simulink model "EFPR_HPT"  (R2024a)
settings: Solver=VariableStepAuto  StartTime=0.0  StopTime=inf  RelTol=1e-3
undefined symbols (not defined in the file): CR, LF
libraries: instrumentseriallib x2, slrealtimeseriallib x1
settings Model: Creator=enrea  LastModifiedBy=enrea

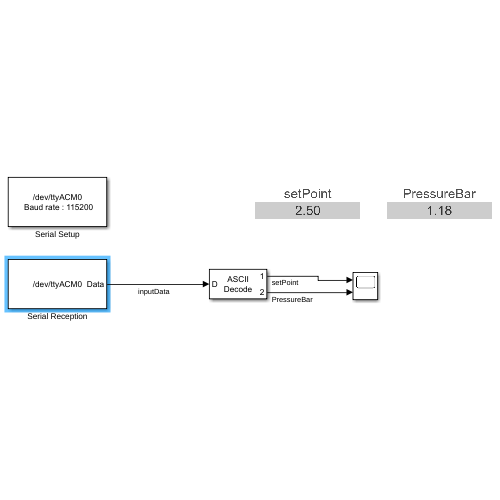
[thumbnail: Simulink's stored preview of the top-level diagram]
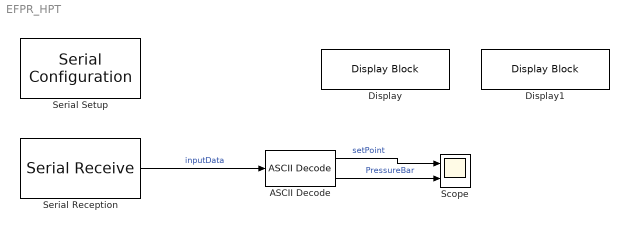
== system EFPR_HPT ==
  ASCII Decode : slrealtimeseriallib/ASCII Decode  format=%f|%f  nvars=2  vartypes={ }
  Display : DisplayBlock  Format=Custom  Transparency=1  FormatString=%.2f
  Display1 : DisplayBlock  Format=Custom  Transparency=1  FormatString=%.2f
  Scope : Scope  NumInputPorts=2
  Serial Reception : instrumentseriallib/Serial Receive  PortSel=/dev/ttyACM0  Port=/dev/ttyACM0  ComPort=/dev/ttyACM0  DataType=int8  SaveDataType=uint8  ToggleHeader=off  Header='S'  ToggleDataSize=on  DataSize=9  ToggleTerminator=on  Terminator=CR/LF ('\r\n')  CustomTerminator='E'  InputFormat=Row major  EnableBlockingMode=on  ActionDataUnavailable=Output last received value  ActionWhenDataUnavailable=Output last received value  CustomValue=0  SampleTime=-1  SimulateUsing=Interpreted execution  BlockInModel=on  aMode=5
      settings: LibrarySourceBlock=mcblib/Protection and Diagnostics/Host Serial Receive
  Serial Setup : instrumentseriallib/Serial Configuration  Priority=-99  PortSel=/dev/ttyACM0  Port=/dev/ttyACM0  ComPort=/dev/ttyACM0  BaudRate=115200  DataBits=8  Parity=none  StopBits=1  ByteOrder=little-endian  FlowControl=none  Timeout=1  SimulateUsing=Interpreted execution  BlockInModel=on  aMode=5
      settings: LibrarySourceBlock=mcblib/Protection and Diagnostics/Host Serial Setup
  wires:
  ASCII Decode/1 -> Scope/1  "setPoint"
  ASCII Decode/2 -> Scope/2  "PressureBar"
  Serial Reception/1 -> ASCII Decode/1  "inputData"
